simulink model "bldc_sixstep_f28069mLaunchPad"  (R2023b)
settings: Solver=FixedStepAuto  StartTime=0.0  StopTime=1.6  RelTol=1e-3  EnableMultiTasking=on
values from neighbouring files (symbols this model uses):
  bldc = mcb_SetPMSMMotorParameters('Teknic2310P')    [bldc_sixstep_f28069mLaunchPad_data.m]    (also in projectData.mat = )
  inverter = mcb_SetInverterParameters('BoostXL-DRV8305')    [bldc_sixstep_f28069mLaunchPad_data.m]    (also in projectData.mat = )
  PI_params = mcb_SetControllerParameters(bldc,inverter,PU_System,T_pwm,2*Ts,Ts_speed)    [bldc_sixstep_f28069mLaunchPad_data.m]    (also in projectData.mat = )
  PWM_frequency = 20e3    (= 20000)    [bldc_sixstep_f28069mLaunchPad_data.m]    (also in projectData.mat)
  target = mcb_SetProcessorDetails('F28069M',PWM_frequency)    [bldc_sixstep_f28069mLaunchPad_data.m]    (also in projectData.mat = )
  Ts = T_pwm    (= 5e-05)    [bldc_sixstep_f28069mLaunchPad_data.m]    (also in projectData.mat)
  Ts_motor_simscape = T_pwm/100    (= 5e-07)    [bldc_sixstep_f28069mLaunchPad_data.m]    (also in projectData.mat)
  Ts_simulink = T_pwm/2    (= 2.5e-05)    [bldc_sixstep_f28069mLaunchPad_data.m]    (also in projectData.mat)
  Ts_speed = 10*Ts    (= 0.0005)    [bldc_sixstep_f28069mLaunchPad_data.m]    (also in projectData.mat)
libraries: nesl_utility x14, fl_lib x9, mcbcontrolslib x7, simulink x6, pil_lib x6, ee_lib x5, slpidlib x4, mcbpositiondecoderlib x4
(part 3 of 3)

== system bldc_sixstep_f28069mLaunchPad/Inverter and Motor/Sensor_Measurements/Halls/Hall State Plant to HW ==
  HallStatePlant : Inport
  Data Type Conversion : DataTypeConversion  OutDataTypeStr=uint8  SaturateOnIntegerOverflow=off  RndMeth=Floor
  If Action Subsystem : Subsystem  TreatAsAtomicUnit=on
  If Action Subsystem1 : Subsystem  TreatAsAtomicUnit=on
  If Action Subsystem2 : Subsystem  TreatAsAtomicUnit=on
  If Action Subsystem3 : Subsystem  TreatAsAtomicUnit=on
  If Action Subsystem4 : Subsystem  TreatAsAtomicUnit=on
  If Action Subsystem5 : Subsystem  TreatAsAtomicUnit=on
  Merge : Merge  Inputs=6
  Switch Case : SwitchCase  CaseConditions={1,5,4,6,2,3}  ShowDefaultCase=off
  HallstateHw : Outport
  wires:
  Merge/1 -> Data Type Conversion/1
  HallStatePlant/1 -> Switch Case/1
  If Action Subsystem3/1(Out1) -> Merge/4
  Switch Case/4 -> If Action Subsystem3/Action
  If Action Subsystem5/1(Out1) -> Merge/6
  Switch Case/1 -> If Action Subsystem/Action
  Switch Case/6 -> If Action Subsystem5/Action
  Switch Case/3 -> If Action Subsystem2/Action
  If Action Subsystem/1(Out1) -> Merge/1
  If Action Subsystem4/1(Out1) -> Merge/5
  Switch Case/5 -> If Action Subsystem4/Action
  If Action Subsystem2/1(Out1) -> Merge/3
  If Action Subsystem1/1(Out1) -> Merge/2
  Switch Case/2 -> If Action Subsystem1/Action
  Data Type Conversion/1 -> HallstateHw/1

== system bldc_sixstep_f28069mLaunchPad/Controller/Subsystem/Input scaling/Hall Feedback/Speed Counter ==
  Hall_State : Inport
  AND : Logic  IconShape=distinctive  AllPortsSameDT=off  OutDataTypeStr=boolean
  Constant1 : Constant
  Constant4 : Constant  OutDataTypeStr=uint32  SampleTime=-1
  Delay : Delay  DelayLength=1  InitialCondition=1  ExternalReset=Level
      settings: InputPortMap=u0,r5
  Detect Change : simulink/Logic and Bit Operations/Detect Change  vinit=0  OutDataTypeStr=boolean
  Enabled Subsystem : Subsystem  TreatAsAtomicUnit=on
  Sum : Sum  Inputs=|++  OutDataTypeStr=uint32  AccumDataTypeStr=uint32  RndMeth=Simplest
  Unit Delay : UnitDelay  InitialCondition=1  SampleTime=-1  HasFrameUpgradeWarning=on
  Previous_Hall_State : Outport
  Speed_Count : Outport  Port=2
  wires:
  Delay/1 -> Unit Delay/1, Sum/2
  Constant4/1 -> Sum/1
  Sum/1 -> Delay/1
  Unit Delay/1 -> Enabled Subsystem/1(In1)
  Detect Change/1 -> Enabled Subsystem/Enable, AND/2
  Enabled Subsystem/1(Speed_Count) -> Speed_Count/1
  Hall_State/1 -> Enabled Subsystem/2(Hall_State), Detect Change/1
  Enabled Subsystem/2(PrevHallState) -> Previous_Hall_State/1
  AND/1 -> Delay/2
  Constant1/1 -> AND/1

== system bldc_sixstep_f28069mLaunchPad/Controller/Subsystem/Input scaling/Hall Feedback/Subsystem ==
  Hall_C : Inport
  Hall_B : Inport  Port=2
  Hall_A : Inport  Port=3
  Shift Arithmetic : ArithShift  BitShiftNumber=2  BitShiftDirection=Left
  Shift Arithmetic1 : ArithShift  BitShiftNumber=1  BitShiftDirection=Left
  Sum : Sum  Inputs=|+++
  HallState : Outport
  wires:
  Shift Arithmetic/1 -> Sum/1
  Shift Arithmetic1/1 -> Sum/2
  Hall_C/1 -> Shift Arithmetic/1
  Hall_A/1 -> Sum/3
  Sum/1 -> HallState/1
  Hall_B/1 -> Shift Arithmetic1/1

== system bldc_sixstep_f28069mLaunchPad/Current control/Input scaling/Hall Feedback/Speed Counter/Enabled Subsystem ==
  In1 : Inport
  Hall_State : Inport  Port=2
  Enable : EnablePort
  Constant4 : Constant  OutDataTypeStr=uint32  SampleTime=-1
  Sum : Sum  Inputs=|++  OutDataTypeStr=uint32  AccumDataTypeStr=uint32  RndMeth=Simplest
  Unit Delay1 : UnitDelay  InitialCondition=1  SampleTime=-1  HasFrameUpgradeWarning=on
  Speed_Count : Outport
  PrevHallState : Outport  Port=2
  wires:
  Sum/1 -> Speed_Count/1
  Constant4/1 -> Sum/2
  In1/1 -> Sum/1
  Hall_State/1 -> Unit Delay1/1
  Unit Delay1/1 -> PrevHallState/1

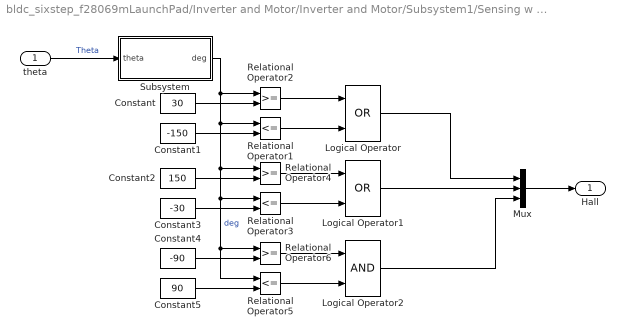
== system bldc_sixstep_f28069mLaunchPad/Inverter and Motor/Inverter and Motor/Subsystem1/Sensing w a/Hall sensor ==
  theta : Inport
  Constant : Constant  Value=30
  Constant1 : Constant  Value=-150
  Constant2 : Constant  Value=150
  Constant3 : Constant  Value=-30
  Constant4 : Constant  Value=-90
  Constant5 : Constant  Value=90
  Logical Operator : Logic  Operator=OR  AllPortsSameDT=off  OutDataTypeStr=boolean
  Logical Operator1 : Logic  Operator=OR  AllPortsSameDT=off  OutDataTypeStr=boolean
  Logical Operator2 : Logic  AllPortsSameDT=off  OutDataTypeStr=boolean
  Mux : Mux  Inputs=3
  Relational Operator1 : RelationalOperator  Operator=<=
  Relational Operator2 : RelationalOperator
  Relational Operator3 : RelationalOperator  Operator=<=
  Relational Operator4 : RelationalOperator
  Relational Operator5 : RelationalOperator  Operator=<=
  Relational Operator6 : RelationalOperator
  Subsystem : Subsystem
  Hall : Outport  VectorParamsAs1DForOutWhenUnconnected=off
  wires:
  theta/1 -> Subsystem/1(theta)  "Theta"
  Constant2/1 -> Relational Operator4/2
  Constant1/1 -> Relational Operator1/2
  Relational Operator4/1 -> Logical Operator1/1
  Constant/1 -> Relational Operator2/2
  Subsystem/1(deg) -> Relational Operator2/1, Relational Operator1/1, Relational Operator6/1, Relational Operator5/1, Relational Operator3/1, Relational Operator4/1  "deg"
  Relational Operator1/1 -> Logical Operator/2
  Relational Operator2/1 -> Logical Operator/1
  Mux/1 -> Hall/1
  Relational Operator3/1 -> Logical Operator1/2
  Constant5/1 -> Relational Operator5/2
  Constant4/1 -> Relational Operator6/2
  Relational Operator6/1 -> Logical Operator2/1
  Relational Operator5/1 -> Logical Operator2/2
  Logical Operator/1 -> Mux/1
  Logical Operator1/1 -> Mux/2
  Logical Operator2/1 -> Mux/3
  Constant3/1 -> Relational Operator3/2

== system bldc_sixstep_f28069mLaunchPad/Inverter and Motor/Sensor_Measurements/Halls/Hall State Plant to HW/If Action Subsystem ==
  Action Port : ActionPort  ActionPortLabel=case [ 1 ]:
  Constant : Constant  Value=bldc.HallSequence(1)  OutDataTypeStr=uint16
  Out1 : Outport
  wires:
  Constant/1 -> Out1/1

== system bldc_sixstep_f28069mLaunchPad/Inverter and Motor/Sensor_Measurements/Halls/Hall State Plant to HW/If Action Subsystem1 ==
  Action Port : ActionPort  ActionPortLabel=case [ 5 ]:
  Constant : Constant  Value=bldc.HallSequence(2)  OutDataTypeStr=uint16
  Out1 : Outport
  wires:
  Constant/1 -> Out1/1

== system bldc_sixstep_f28069mLaunchPad/Inverter and Motor/Sensor_Measurements/Halls/Hall State Plant to HW/If Action Subsystem2 ==
  Action Port : ActionPort  ActionPortLabel=case [ 4 ]:
  Constant : Constant  Value=bldc.HallSequence(3)  OutDataTypeStr=uint16
  Out1 : Outport
  wires:
  Constant/1 -> Out1/1

== system bldc_sixstep_f28069mLaunchPad/Inverter and Motor/Sensor_Measurements/Halls/Hall State Plant to HW/If Action Subsystem3 ==
  Action Port : ActionPort  ActionPortLabel=case [ 6 ]:
  Constant : Constant  Value=bldc.HallSequence(4)  OutDataTypeStr=uint16
  Out1 : Outport
  wires:
  Constant/1 -> Out1/1

== system bldc_sixstep_f28069mLaunchPad/Inverter and Motor/Sensor_Measurements/Halls/Hall State Plant to HW/If Action Subsystem4 ==
  Action Port : ActionPort  ActionPortLabel=case [ 2 ]:
  Constant : Constant  Value=bldc.HallSequence(5)  OutDataTypeStr=uint16
  Out1 : Outport
  wires:
  Constant/1 -> Out1/1

== system bldc_sixstep_f28069mLaunchPad/Inverter and Motor/Sensor_Measurements/Halls/Hall State Plant to HW/If Action Subsystem5 ==
  Action Port : ActionPort  ActionPortLabel=case [ 3 ]:
  Constant : Constant  Value=bldc.HallSequence(6)  OutDataTypeStr=uint16
  Out1 : Outport
  wires:
  Constant/1 -> Out1/1

== system bldc_sixstep_f28069mLaunchPad/Controller/Subsystem/Input scaling/Hall Feedback/Speed Counter/Enabled Subsystem ==
  In1 : Inport
  Hall_State : Inport  Port=2
  Enable : EnablePort
  Constant4 : Constant  OutDataTypeStr=uint32  SampleTime=-1
  Sum : Sum  Inputs=|++  OutDataTypeStr=uint32  AccumDataTypeStr=uint32  RndMeth=Simplest
  Unit Delay1 : UnitDelay  InitialCondition=1  SampleTime=-1  HasFrameUpgradeWarning=on
  Speed_Count : Outport
  PrevHallState : Outport  Port=2
  wires:
  Sum/1 -> Speed_Count/1
  Constant4/1 -> Sum/2
  In1/1 -> Sum/1
  Hall_State/1 -> Unit Delay1/1
  Unit Delay1/1 -> PrevHallState/1

== system bldc_sixstep_f28069mLaunchPad/Inverter and Motor/Inverter and Motor/Subsystem1/Sensing w a/Hall sensor/Subsystem ==
  theta : Inport
  Trigonometric Function : Trigonometry  Operator=sincos
  Trigonometric Function2 : Trigonometry  Operator=atan2
  mech->elec : Gain  Gain=bldc.p
  rad->deg : Gain  Gain=180/pi  SaturateOnIntegerOverflow=on  OutDataTypeStr=Inherit: Same as input  ParamDataTypeStr=Inherit: Same as input
  deg : Outport  VectorParamsAs1DForOutWhenUnconnected=off
  wires:
  mech->elec/1 -> Trigonometric Function/1
  Trigonometric Function/2 -> Trigonometric Function2/2
  rad->deg/1 -> deg/1
  theta/1 -> mech->elec/1
  Trigonometric Function/1 -> Trigonometric Function2/1
  Trigonometric Function2/1 -> rad->deg/1
